simulink model "PMSM_speed"  (Simulink 8.0)
settings: Solver=ode45  StartTime=0.0  StopTime=0.05  RelTol=1e-3
InitFcn:
  | clc;
  | clear;
  | Ra=2.875;
  | Lq=8.5e-3;
  | Ld=8.5e-3;
  | phim=0.175;
  | p=8;
  | J=8e-4;
  | Bm=0;
StopFcn:
  | clc;
libraries: simulink x1
Description:
  | This demonstration illustrates the use of the PMSM in a closed-loop
  | speed and current control on a 1.1 kW  3000 rpm industrial motor.
  | 
  | A three-phase motor rated 1.1 KW, 220 V, 3000 rpm is fed by a PWM inverter. In this demo,
  | the whole system is buildt entirely with standard Simulink blocks (without resort to blocksets).
  | The initial load torque is set at the nominal value (3 N.m) and steps down to 1 N.m at t=0.03s.
  | Two control loops are used: the inner loop regulates the currents and the outer loop controls
  | the speed.
  | Field orientation is obtained by setting  id_ref to zero. The torque command iq_ref is derived
  | from the  speed controller.
settings Model: Creator=AbdulRahman  LastModifiedBy=AbdulRahman

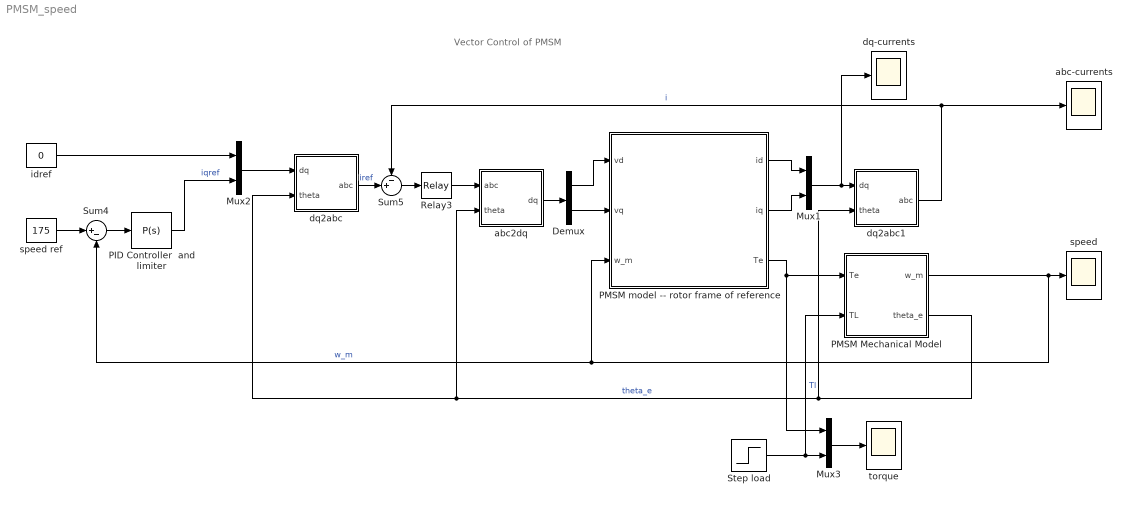
== system PMSM_speed ==
  note: Vector Control of PMSM
  Demux : Demux  Outputs=2
  Mux1 : Mux  Inputs=2
  Mux2 : Mux  Inputs=2
  Mux3 : Mux  Inputs=2
  PID Controller  and limiter : simulink/Continuous/PID Controller  Controller=P  TimeDomain=Continuous-time  SampleTime=1  IntegratorMethod=Forward Euler  FilterMethod=Forward Euler  Form=Parallel  P=10  I=1  D=0  N=100  InitialConditionSource=internal  InitialConditionForIntegrator=0  InitialConditionForFilter=0  ExternalReset=none  LimitOutput=on  UpperSaturationLimit=10  LowerSaturationLimit=-10  LinearizeAsGain=on  AntiWindupMode=none  Kb=1  TrackingMode=off  Kt=1  PParamMin=[]  PParamMax=[]  IParamMin=[]  IParamMax=[]  DParamMin=[]  DParamMax=[]  NParamMin=[]  NParamMax=[]  KbParamMin=[]  KbParamMax=[]  KtParamMin=[]  KtParamMax=[]  POutMin=[]  POutMax=[]  IOutMin=[]  IOutMax=[]  DOutMin=[]  DOutMax=[]  NOutMin=[]  NOutMax=[]  KbOutMin=[]  KbOutMax=[]  KtOutMin=[]  KtOutMax=[]  IntegratorOutMin=[]  IntegratorOutMax=[]  FilterOutMin=[]  FilterOutMax=[]  SumOutMin=[]  SumOutMax=[]  SumI1OutMin=[]  SumI1OutMax=[]  SumI2OutMin=[]  SumI2OutMax=[]  SumI3OutMin=[]  SumI3OutMax=[]  SumDOutMin=[]  SumDOutMax=[]  SaturationOutMin=[]  SaturationOutMax=[]  IntegratorContinuousStateAttributes=''  IntegratorStateMustResolveToSignalObject=off  IntegratorRTWStateStorageClass=Auto  FilterContinuousStateAttributes=''  FilterStateMustResolveToSignalObject=off  FilterRTWStateStorageClass=Auto
  PMSM Mechanical Model : Subsystem
  "PMSM model -- rotor frame of reference" : Subsystem
  Relay3 : Relay  OnSwitchValue=0.1  OffSwitchValue=-0.1  OnOutputValue=155  OffOutputValue=-155
  Step load : Step  Time=0.03  Before=3  SampleTime=0
  Sum4 : Sum  Inputs=|+-  SaturateOnIntegerOverflow=on  InputSameDT=on  OutDataTypeStr=Inherit: Same as first input
  Sum5 : Sum  Inputs=-+|  SaturateOnIntegerOverflow=on  InputSameDT=on  OutDataTypeStr=Inherit: Same as first input
  abc-currents : Scope
      settings: TimeRange=0.05  YMin=-15  YMax=15  MaxDataPoints=25000
  abc2dq : Subsystem
  dq-currents : Scope
      settings: TimeRange=0.05  YMin=-2  YMax=12  SaveName=ScopeData3  MaxDataPoints=25000
  dq2abc : Subsystem
  dq2abc1 : Subsystem
  idref : Constant  Value=0
  speed : Scope
      settings: TimeRange=0.05  YMin=-50  YMax=200  MaxDataPoints=25000
  speed ref : Constant  Value=175
  torque : Scope
      settings: TimeRange=0.05  YMin=0  YMax=12  SaveName=ScopeData2  MaxDataPoints=25000
  wires:
  speed ref/1 -> Sum4/1
  Sum4/1 -> PID Controller  and limiter/1
  PID Controller  and limiter/1 -> Mux2/2  "iqref"
  idref/1 -> Mux2/1
  Mux1/1 -> dq2abc1/1(dq), dq-currents/1
  "PMSM model -- rotor frame of reference"/1(id) -> Mux1/1
  "PMSM model -- rotor frame of reference"/2(iq) -> Mux1/2
  dq2abc/1(abc) -> Sum5/2  "iref"
  dq2abc1/1(abc) -> Sum5/1, abc-currents/1  "i"
  Sum5/1 -> Relay3/1
  Relay3/1 -> abc2dq/1(abc)
  abc2dq/1(dq) -> Demux/1
  Demux/1 -> "PMSM model -- rotor frame of reference"/1(vd)
  "PMSM model -- rotor frame of reference"/3(Te) -> Mux3/1, PMSM Mechanical Model/1(Te)
  Step load/1 -> PMSM Mechanical Model/2(TL), Mux3/2  "Tl"
  Mux3/1 -> torque/1
  Demux/2 -> "PMSM model -- rotor frame of reference"/2(vq)
  Mux2/1 -> dq2abc/1(dq)
  PMSM Mechanical Model/1(w_m) -> "PMSM model -- rotor frame of reference"/3(w_m), Sum4/2, speed/1  "w_m"
  PMSM Mechanical Model/2(theta_e) -> dq2abc1/2(theta), abc2dq/2(theta), dq2abc/2(theta)  "theta_e"

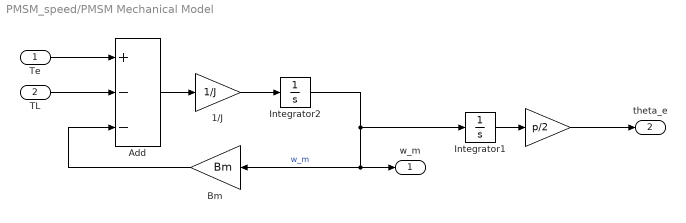
== system PMSM_speed/PMSM Mechanical Model ==
  Te : Inport
  TL : Inport  Port=2
  "  " : Gain  Gain=p/2  OutDataTypeStr=Inherit: Same as input  ParamDataTypeStr=Inherit: Same as input
  1/J : Gain  Gain=1/J  OutDataTypeStr=Inherit: Same as input  ParamDataTypeStr=Inherit: Same as input
  Add : Sum  Inputs=+--
  Bm : Gain  Gain=Bm  SaturateOnIntegerOverflow=on  OutDataTypeStr=Inherit: Same as input  ParamDataTypeStr=Inherit: Same as input
  Integrator1 : Integrator
  Integrator2 : Integrator
  w_m : Outport
  theta_e : Outport  Port=2
  wires:
  "  "/1 -> theta_e/1
  1/J/1 -> Integrator2/1
  Integrator2/1 -> Bm/1, w_m/1, Integrator1/1  "w_m"
  Add/1 -> 1/J/1
  Integrator1/1 -> "  "/1
  Te/1 -> Add/1
  TL/1 -> Add/2
  Bm/1 -> Add/3

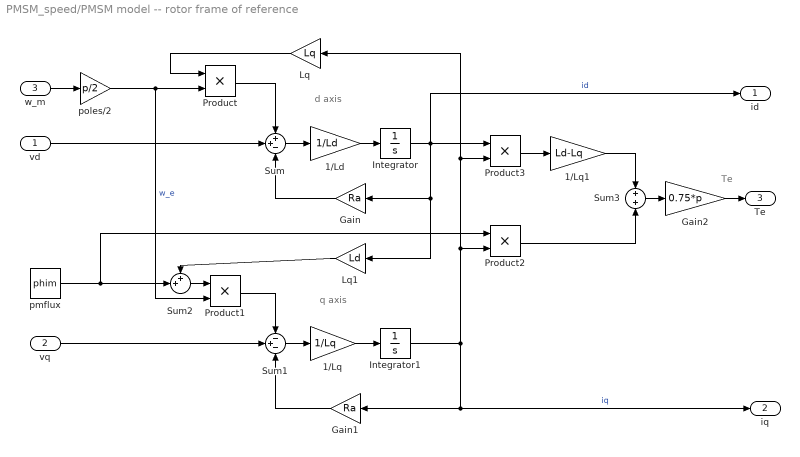
== system PMSM_speed/PMSM model -- rotor frame of reference ==
  note: q axis
  note: d axis
  note: Te
  vd : Inport
  vq : Inport  Port=2
  w_m : Inport  Port=3
  1/Ld : Gain  Gain=1/Ld  SaturateOnIntegerOverflow=on  OutDataTypeStr=Inherit: Same as input  ParamDataTypeStr=Inherit: Same as input
  1/Lq : Gain  Gain=1/Lq  SaturateOnIntegerOverflow=on  OutDataTypeStr=Inherit: Same as input  ParamDataTypeStr=Inherit: Same as input
  1/Lq1 : Gain  Gain=Ld-Lq  SaturateOnIntegerOverflow=on  OutDataTypeStr=Inherit: Same as input  ParamDataTypeStr=Inherit: Same as input
  Gain : Gain  Gain=Ra  SaturateOnIntegerOverflow=on  OutDataTypeStr=Inherit: Same as input  ParamDataTypeStr=Inherit: Same as input
  Gain1 : Gain  Gain=Ra  SaturateOnIntegerOverflow=on  OutDataTypeStr=Inherit: Same as input  ParamDataTypeStr=Inherit: Same as input
  Gain2 : Gain  Gain=0.75*p  SaturateOnIntegerOverflow=on  OutDataTypeStr=Inherit: Same as input  ParamDataTypeStr=Inherit: Same as input
  Integrator : Integrator
  Integrator1 : Integrator
  Lq : Gain  Gain=Lq  SaturateOnIntegerOverflow=on  OutDataTypeStr=Inherit: Same as input  ParamDataTypeStr=Inherit: Same as input
  Lq1 : Gain  Gain=Ld  SaturateOnIntegerOverflow=on  OutDataTypeStr=Inherit: Same as input  ParamDataTypeStr=Inherit: Same as input
  Product{,1..3} (4 alike) : Product  SaturateOnIntegerOverflow=on  InputSameDT=on  OutDataTypeStr=Inherit: Same as first input
  Sum : Sum  Inputs=++-  SaturateOnIntegerOverflow=on  InputSameDT=on  OutDataTypeStr=Inherit: Same as first input
  Sum1 : Sum  Inputs=-+-  SaturateOnIntegerOverflow=on  InputSameDT=on  OutDataTypeStr=Inherit: Same as first input
  Sum2 : Sum  Inputs=++|  SaturateOnIntegerOverflow=on  InputSameDT=on  OutDataTypeStr=Inherit: Same as first input
  Sum3 : Sum  SaturateOnIntegerOverflow=on  InputSameDT=on  OutDataTypeStr=Inherit: Same as first input
  pmflux : Constant  Value=phim
  poles/2 : Gain  Gain=p/2  SaturateOnIntegerOverflow=on  OutDataTypeStr=Inherit: Same as input  ParamDataTypeStr=Inherit: Same as input
  id : Outport
  iq : Outport  Port=2
  Te : Outport  Port=3
  wires:
  Gain/1 -> Sum/3
  vq/1 -> Sum1/2
  Gain1/1 -> Sum1/3
  Integrator/1 -> Gain/1, Lq1/1, Product3/1, id/1  "id"
  Product1/1 -> Sum1/1
  Product/1 -> Sum/1
  Lq/1 -> Product/1
  vd/1 -> Sum/2
  Sum1/1 -> 1/Lq/1
  Sum/1 -> 1/Ld/1
  Sum3/1 -> Gain2/1
  Gain2/1 -> Te/1
  w_m/1 -> poles/2/1
  poles/2/1 -> Product/2, Product1/2  "w_e"
  1/Ld/1 -> Integrator/1
  1/Lq/1 -> Integrator1/1
  Integrator1/1 -> Product2/2, Product3/2, Lq/1, Gain1/1, iq/1  "iq"
  Sum2/1 -> Product1/1
  pmflux/1 -> Sum2/2, Product2/1
  Product3/1 -> 1/Lq1/1
  Product2/1 -> Sum3/2
  1/Lq1/1 -> Sum3/1
  Lq1/1 -> Sum2/1

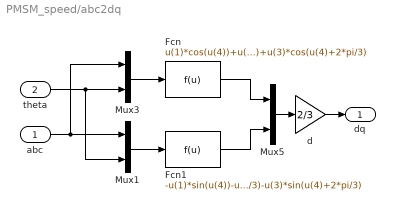
== system PMSM_speed/abc2dq ==
  abc : Inport
  theta : Inport  Port=2
  Fcn : Fcn  Expr=u(1)*cos(u(4))+u(2)*cos(u(4)-2*pi/3)+u(3)*cos(u(4)+2*pi/3)
  Fcn1 : Fcn  Expr=-u(1)*sin(u(4))-u(2)*sin(u(4)-2*pi/3)-u(3)*sin(u(4)+2*pi/3)
  Mux1 : Mux  Inputs=2
  Mux3 : Mux  Inputs=2
  Mux5 : Mux  Inputs=2
  d : Gain  Gain=2/3  OutDataTypeStr=Inherit: Same as input  ParamDataTypeStr=Inherit: Same as input
  dq : Outport
  wires:
  Mux3/1 -> Fcn/1
  Fcn/1 -> Mux5/1
  Mux5/1 -> d/1
  Mux1/1 -> Fcn1/1
  Fcn1/1 -> Mux5/2
  abc/1 -> Mux1/1, Mux3/1
  theta/1 -> Mux3/2, Mux1/2
  d/1 -> dq/1

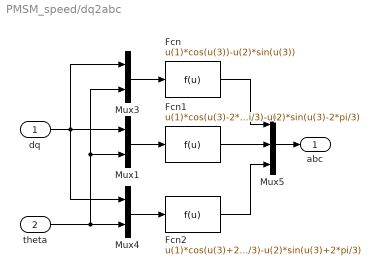
== system PMSM_speed/dq2abc ==
  dq : Inport
  theta : Inport  Port=2
  Fcn : Fcn  Expr=u(1)*cos(u(3))-u(2)*sin(u(3))
  Fcn1 : Fcn  Expr=u(1)*cos(u(3)-2*pi/3)-u(2)*sin(u(3)-2*pi/3)
  Fcn2 : Fcn  Expr=u(1)*cos(u(3)+2*pi/3)-u(2)*sin(u(3)+2*pi/3)
  Mux1 : Mux  Inputs=2
  Mux3 : Mux  Inputs=2
  Mux4 : Mux  Inputs=2
  Mux5 : Mux  Inputs=3
  abc : Outport
  wires:
  Mux3/1 -> Fcn/1
  Mux4/1 -> Fcn2/1
  dq/1 -> Mux3/1, Mux4/1, Mux1/1
  Fcn/1 -> Mux5/1
  Mux5/1 -> abc/1
  Mux1/1 -> Fcn1/1
  Fcn1/1 -> Mux5/2
  Fcn2/1 -> Mux5/3
  theta/1 -> Mux4/2, Mux3/2, Mux1/2

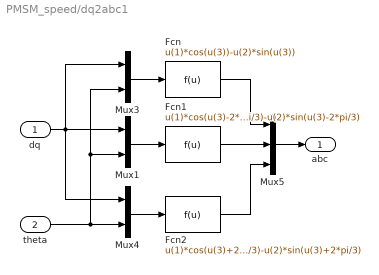
== system PMSM_speed/dq2abc1 ==
  dq : Inport
  theta : Inport  Port=2
  Fcn : Fcn  Expr=u(1)*cos(u(3))-u(2)*sin(u(3))
  Fcn1 : Fcn  Expr=u(1)*cos(u(3)-2*pi/3)-u(2)*sin(u(3)-2*pi/3)
  Fcn2 : Fcn  Expr=u(1)*cos(u(3)+2*pi/3)-u(2)*sin(u(3)+2*pi/3)
  Mux1 : Mux  Inputs=2
  Mux3 : Mux  Inputs=2
  Mux4 : Mux  Inputs=2
  Mux5 : Mux  Inputs=3
  abc : Outport
  wires:
  theta/1 -> Mux1/2, Mux3/2, Mux4/2
  Fcn2/1 -> Mux5/3
  Fcn1/1 -> Mux5/2
  Mux1/1 -> Fcn1/1
  Mux5/1 -> abc/1
  Fcn/1 -> Mux5/1
  Mux4/1 -> Fcn2/1
  Mux3/1 -> Fcn/1
  dq/1 -> Mux3/1, Mux1/1, Mux4/1
